simulink model "buildover_fullstatemachine"  (R2023a)
settings: Solver=FixedStepDiscrete  StartTime=0.0  StopTime=inf  FixedStep=0.001  RelTol=1e-3  EnableMultiTasking=on
undefined symbols (not defined in the file): dev, DiscIntNeverNeededParam, Main, output, pwm_output0, timestamp
libraries: simulink x15, px4uORBlib x7, robotcorelib x2, dspsigops x2, px4lib x1, px4Sensorslib x1, sharedtransform x1
settings Model: ExtModeTrigDuration=10  Creator=Kristan  LastModifiedBy=Kristan
settings SolverCC: PositivePriorityOrder=on  AutoInsertRateTranBlk=on
settings OptimizationCC: StrengthReduction=on  MemcpyThreshold=256  PassReuseOutputArgsAs=Individual arguments  ZeroExternalMemoryAtStartup=off  ZeroInternalMemoryAtStartup=off  MaxStackSize=128  OptimizeBlockOrder=speed  OptimizationPriority=Speed  OptimizationCustomize=off  MultiThreadedLoops=on  EfficientTunableParamExpr=on
settings DebuggingCC: ParameterTunabilityLossMsg=error  UnderSpecifiedDimensionMsg=warning
settings HardwareCC: ProdBitPerPointer=32  ProdBitPerSizeT=32  ProdBitPerPtrDiffT=32  ProdLargestAtomicInteger=Long  ProdLargestAtomicFloat=Double  ProdWordSize=32  ProdLongLongMode=on  ProdHWDeviceType=ARM Compatible->ARM Cortex
settings SFSimCC: MATLABDynamicMemAlloc=off  SimTargetLang=C++
settings RTWCC: Description=Embedded Coder  SystemTargetFile=ert.tlc  HardwareBoard=PX4 Pixhawk 6x  TLCOptions="-aInlineSetEventsForThisBaseRateFcn=TLC_FALSE -aSuppressMultiTaskScheduler=TLC_FALSE  -aRateBasedStepFcn=0"  TemplateMakefile=ert_default_tmf  GenerateReport=on  Toolchain=GNU Tools for PX4 Autopilots  LaunchReport=on  CodeProfilingSaveOptions=AllData  TargetLang=C++  GenerateCodeMetricsReport=on
settings CodeAppCC: GenerateComments=off  IgnoreCustomStorageClasses=off  OperatorAnnotations=on  SimulinkDataObjDesc=on  SFDataObjDesc=on  SimulinkBlockComments=off
settings ERTTargetCC: ExtModeTransport=3  ExtModeStaticAlloc=on  ExtModeStaticAllocSize=1024  ExtModeMexFile=ext_xcp  ExtModeIntrfLevel=Level2 - Open

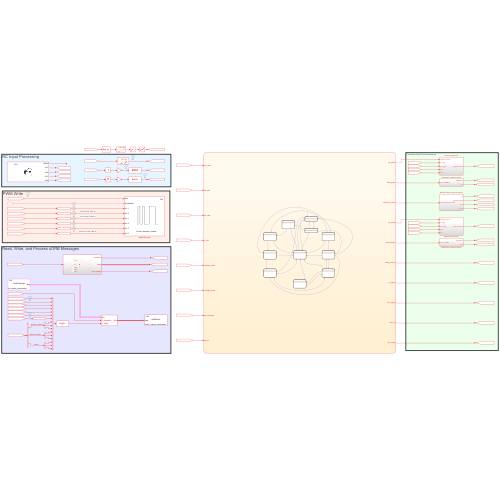
[thumbnail: Simulink's stored preview of the top-level diagram]
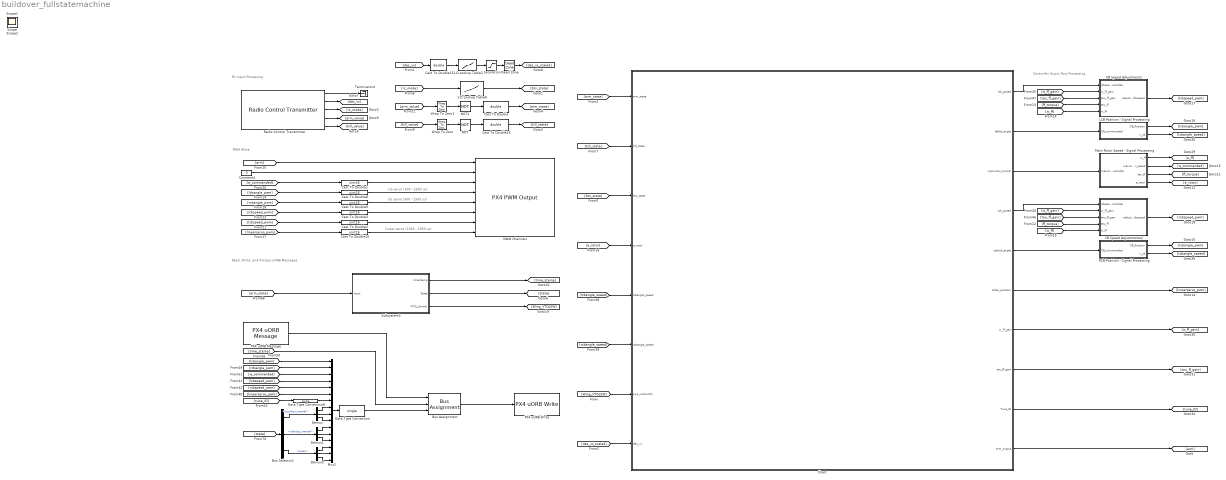
== system buildover_fullstatemachine ==
  note: Controller Ouput Post Processing
  note: PWM Write
  note: RC Input Processing
  note: Read, Write, and Process uORB Messages
  note: rcb servo (500 - 2500 us)
  note: lcb servo (500 - 2500 us)
  note: linear servo (1050 - 1950 us)
  1-D Lookup Table1 : Lookup_n-D  NumberOfTableDimensions=1  BreakpointsForDimension1=linspace(982,2006,2)  Table=linspace(-5,5,2)  InternalRulePriority=Speed  RndMeth=Simplest
  1-D Lookup Table6 : Lookup_n-D  NumberOfTableDimensions=1  BreakpointsForDimension1=[0, 1050, 1150, 1350, 1515, 1660, 1850]  Table=[1,2,3,4,5,6,7]  InterpMethod=Flat  InternalRulePriority=Speed  RndMeth=Simplest
  Bus Assignment : BusAssignment  AssignedSignals=timestamp,output
  Bus Selector1 : BusSelector  OutputSignals=position_inertial,velocity_inertial,euler
  CB Speed Adjustments : Subsystem
  CB Speed Adjustments2 : Subsystem
  Cast To Double : DataTypeConversion  OutDataTypeStr=double  SaturateOnIntegerOverflow=off  RndMeth=Floor
  Cast To Double{1..3,8..10} (6 alike) : DataTypeConversion  OutDataTypeStr=uint16  SaturateOnIntegerOverflow=off  RndMeth=Floor
  Cast To Double15 : DataTypeConversion  OutDataTypeStr=double  SaturateOnIntegerOverflow=off  RndMeth=Floor
  Cast To Double16 : DataTypeConversion  OutDataTypeStr=double  SaturateOnIntegerOverflow=off  RndMeth=Floor
  Chart : Stateflow chart  TreatAsAtomicUnit=on
  Constant4 : Constant  Value=0  OutDataTypeStr=boolean
  Data Type Conversion : DataTypeConversion  OutDataTypeStr=single  SaturateOnIntegerOverflow=off  RndMeth=Floor
  Data Type Conversion8 : DataTypeConversion  OutDataTypeStr=double  SaturateOnIntegerOverflow=off  RndMeth=Floor
  Dead Zone : DeadZone  LowerValue=-0.1  UpperValue=0.1
  Demux : Demux  Outputs=3
  Demux1 : Demux  Outputs=3
  Demux3 : Demux  Outputs=3
  LCB Position - Signal Processing : Subsystem
  MAIN Channels : px4lib/PX4 PWM Output  pwmDevice=Main (/dev/pwm_output0)  pwmChannel1_=on  pwmChannel2_=on  pwmChannel3_=on  pwmChannel4_=on  pwmChannel5_=on  pwmChannel6_=on  pwmChannel7_=off  pwmChannel8_=off  forceTerminateFailsafe=off  outputErrorStatus=off
  Main Rotor Speed - Signal Processing : Subsystem
  Mux2 : Mux  Inputs=16
  NOT : Logic  Operator=NOT  IconShape=distinctive  AllPortsSameDT=off  OutDataTypeStr=boolean
  NOT1 : Logic  Operator=NOT  IconShape=distinctive  AllPortsSameDT=off  OutDataTypeStr=boolean
  PX4 uORB Message : px4uORBlib/PX4 uORB Message  uORBTopic=actuator_outputs_commanded  SampleTime=inf  selectInstance=actuator_outputs_commanded
  PX4 uORB Write : px4uORBlib/PX4 uORB Write  uORBTopic=actuator_outputs_commanded  selectInstance=actuator_outputs_commanded  MessageQueueLen=1
  RCB Position - Signal Processing : Subsystem
  Radio Control Transmitter : px4Sensorslib/Radio Control Transmitter  channel1=off  channel2=off  channel3=on  channel4=off  channel5=off  channel6=on  channel7=on  channel8=on  channel_count=off  rssi=off  rc_input_source=off  timestamp_last_signal=off  time_stamp=off  sampleTime=-1  BlockingMode=off  BlockTimeout=5
  Saturation : Saturate  UpperLimit=5  LowerLimit=-5
  Subsystem3 : Subsystem
  Terminator4 : Terminator
  Wrap To Zero : simulink/Discontinuities/Wrap To Zero  Threshold=1500
  Wrap To Zero1 : simulink/Discontinuities/Wrap To Zero  Threshold=1500
  Scope : Scope
  Scope1 : Scope
  Scope2 : Scope
  wires:
  Radio Control Transmitter/5 -> [kill_value]
  Radio Control Transmitter/3 -> [rc_mode]
  Radio Control Transmitter/4 -> [arm_value]
  [btn_state] -> Chart/3(btn_state)
  [arm_state] -> Chart/1(arm_state)
  [kill_state] -> Chart/2(kill_state)
  [a_rotor] -> Chart/4(a_rotor)
  Chart/6(slider_position) -> [linearservo_pwm]
  Radio Control Transmitter/1 -> Terminator4/1
  1-D Lookup Table6/1 -> [btn_state]
  [arm_value] -> Wrap To Zero1/1
  Wrap To Zero1/1 -> NOT1/1
  [kill_value] -> Wrap To Zero/1
  [rc_mode] -> 1-D Lookup Table6/1
  Wrap To Zero/1 -> NOT/1
  Cast To Double16/1 -> [kill_state]
  NOT/1 -> Cast To Double16/1
  NOT1/1 -> Cast To Double/1
  Chart/7(w_ff_gain) -> [w_ff_gain]
  Chart/8(tau_ff_gain) -> [tau_ff_gain]
  Chart/3(mainrotor_control) -> Main Rotor Speed - Signal Processing/1(mainmotor_speed_controller)
  Main Rotor Speed - Signal Processing/1(w_ff) -> [w_ff]
  Main Rotor Speed - Signal Processing/2(mainmotor_speed) -> [w_commanded]
  Main Rotor Speed - Signal Processing/3(tau_ff) -> [ff_torque]
  Main Rotor Speed - Signal Processing/4(a_rotor) -> [a_rotor]
  Chart/1(lcb_speed) -> CB Speed Adjustments/1(lcbspeed_controller)
  [w_ff_gain] -> CB Speed Adjustments/2(w_ff_gain)
  [tau_ff_gain] -> CB Speed Adjustments/3(tau_ff_gain)
  [ff_torque] -> CB Speed Adjustments/4(tau_ff)
  [w_ff] -> CB Speed Adjustments/5(w_ff)
  Chart/4(rcb_speed) -> CB Speed Adjustments2/1(rcbspeed_controller)
  [w_ff_gain] -> CB Speed Adjustments2/2(w_ff_gain)
  [tau_ff_gain] -> CB Speed Adjustments2/3(tau_ff_gain)
  [ff_torque] -> CB Speed Adjustments2/4(tau_ff)
  [w_ff] -> CB Speed Adjustments2/5(w_ff)
  Chart/9(Tune_ID) -> [tune_ID]
  Chart/2(leftcb_angle) -> LCB Position - Signal Processing/1(CB_commanded)
  LCB Position - Signal Processing/1(CB_Position) -> [lcbangle_pwm]
  LCB Position - Signal Processing/2(v_cb) -> [lcbangle_speed]
  Chart/5(rightcb_angle) -> RCB Position - Signal Processing/1(CB_commanded)
  RCB Position - Signal Processing/1(CB_Position) -> [rcbangle_pwm]
  RCB Position - Signal Processing/2(v_cb) -> [rcbangle_speed]
  [lcbangle_speed] -> Chart/5(lcbangle_speed)
  [rcbangle_speed] -> Chart/6(rcbangle_speed)
  Cast To Double/1 -> [arm_state]
  PX4 uORB Message/1 -> Bus Assignment/1
  Bus Assignment/1 -> PX4 uORB Write/1
  [tune_ID] -> Data Type Conversion8/1
  Mux2/1 -> Data Type Conversion/1
  [rcbangle_pwm] -> Mux2/2
  [lcbangle_pwm] -> Mux2/1
  Chart/10(arm_output) -> [arm]
  [time_stamp] -> Bus Assignment/2
  CB Speed Adjustments/1(adjusted_lcbspeed) -> [lcbspeed_pwm]
  CB Speed Adjustments2/1(adjusted_rcbspeed) -> [rcbspeed_pwm]
  Subsystem3/2(State) -> [state]
  [arm_state] -> Subsystem3/1(Input)
  Subsystem3/1(timestamp) -> [time_stamp]
  [state] -> Bus Selector1/1
  Bus Selector1/2 -> Demux1/1  "<velocity_inertial>"
  Bus Selector1/3 -> Demux3/1  "<euler>"
  Bus Selector1/1 -> Demux/1  "<position_inertial>"
  Data Type Conversion/1 -> Bus Assignment/3
  Cast To Double8/1 -> MAIN Channels/4
  Cast To Double10/1 -> MAIN Channels/8
  Cast To Double2/1 -> MAIN Channels/7
  Cast To Double3/1 -> MAIN Channels/6
  Cast To Double1/1 -> MAIN Channels/3
  Cast To Double9/1 -> MAIN Channels/5
  [w_commanded] -> Cast To Double1/1
  Constant4/1 -> MAIN Channels/2
  [lcbspeed_pwm] -> Cast To Double2/1
  [rcbangle_pwm] -> Cast To Double9/1
  [rcbspeed_pwm] -> Cast To Double3/1
  [arm] -> MAIN Channels/1
  [linearservo_pwm] -> Cast To Double10/1
  [lcbangle_pwm] -> Cast To Double8/1
  [w_commanded] -> Mux2/3
  [lcbspeed_pwm] -> Mux2/4
  [rcbspeed_pwm] -> Mux2/5
  [linearservo_pwm] -> Mux2/6
  Data Type Conversion8/1 -> Mux2/7
  Demux3/3 -> Mux2/16
  Demux3/2 -> Mux2/15
  Demux3/1 -> Mux2/14
  Demux1/3 -> Mux2/13
  Demux1/2 -> Mux2/12
  Demux1/1 -> Mux2/11
  Demux/3 -> Mux2/10
  Demux/2 -> Mux2/9
  Demux/1 -> Mux2/8
  Subsystem3/3(VTOL_Switch) -> [Wing_VTOLSW]
  [Wing_VTOLSW] -> Chart/7(px4_vtolswitch)
  Radio Control Transmitter/2 -> [des_vx]
  Dead Zone/1 -> [des_vx_scaled]
  Saturation/1 -> Dead Zone/1
  1-D Lookup Table1/1 -> Saturation/1
  Cast To Double15/1 -> 1-D Lookup Table1/1
  [des_vx] -> Cast To Double15/1
  [des_vx_scaled] -> Chart/8(des_vx)

== system buildover_fullstatemachine/CB Speed Adjustments ==
  lcbspeed_controller : Inport
  w_ff_gain : Inport  Port=2
  tau_ff_gain : Inport  Port=3
  tau_ff : Inport  Port=4
  w_ff : Inport  Port=5
  1-D Lookup Table4 : Lookup_n-D  NumberOfTableDimensions=1  BreakpointsForDimension1=linspace(0,3300,2)  Table=linspace(1000,2000,2)  InternalRulePriority=Speed  RndMeth=Simplest
  Add1 : Sum
  Constant2 : Constant  Value=0  OutDataTypeStr=double
  Gain11 : Gain  Gain=0.018
  Gain7 : Gain  Gain=1600
  Product : Product
  Product2 : Product
  Saturation : Saturate  UpperLimit=2000  LowerLimit=1000
  Square1 : Math  Operator=square
  Sum4 : Sum  Inputs=|++
  Sum5 : Sum  Inputs=|++
  adjusted_lcbspeed : Outport
  wires:
  w_ff/1 -> Square1/1
  w_ff_gain/1 -> Product/1
  Product/1 -> Sum4/2
  tau_ff_gain/1 -> Product2/1
  Gain11/1 -> Product/2
  Square1/1 -> Gain11/1
  Product2/1 -> Sum5/2
  Sum4/1 -> 1-D Lookup Table4/1
  tau_ff/1 -> Product2/2
  Sum5/1 -> Sum4/1
  Saturation/1 -> adjusted_lcbspeed/1
  1-D Lookup Table4/1 -> Saturation/1
  Constant2/1 -> Add1/1
  Gain7/1 -> Add1/2
  lcbspeed_controller/1 -> Gain7/1
  Add1/1 -> Sum5/1

== system buildover_fullstatemachine/CB Speed Adjustments2 ==
  rcbspeed_controller : Inport
  w_ff_gain : Inport  Port=2
  tau_ff_gain : Inport  Port=3
  tau_ff : Inport  Port=4
  w_ff : Inport  Port=5
  1-D Lookup Table4 : Lookup_n-D  NumberOfTableDimensions=1  BreakpointsForDimension1=linspace(0,3300,2)  Table=linspace(1000,2000,2)  InternalRulePriority=Speed  RndMeth=Simplest
  Add1 : Sum
  Constant2 : Constant  Value=0  OutDataTypeStr=double
  Gain11 : Gain  Gain=0.018
  Gain6 : Gain  Gain=1600
  Product : Product
  Product2 : Product
  Saturation1 : Saturate  UpperLimit=2000  LowerLimit=1000
  Square1 : Math  Operator=square
  Sum4 : Sum  Inputs=|++
  Sum5 : Sum  Inputs=|++
  adjusted_rcbspeed : Outport
  wires:
  w_ff/1 -> Square1/1
  Sum5/1 -> Sum4/1
  w_ff_gain/1 -> Product/1
  Product/1 -> Sum4/2
  tau_ff_gain/1 -> Product2/1
  Gain11/1 -> Product/2
  Square1/1 -> Gain11/1
  Product2/1 -> Sum5/2
  tau_ff/1 -> Product2/2
  1-D Lookup Table4/1 -> Saturation1/1
  Sum4/1 -> 1-D Lookup Table4/1
  Saturation1/1 -> adjusted_rcbspeed/1
  Constant2/1 -> Add1/1
  Gain6/1 -> Add1/2
  Add1/1 -> Sum5/1
  rcbspeed_controller/1 -> Gain6/1

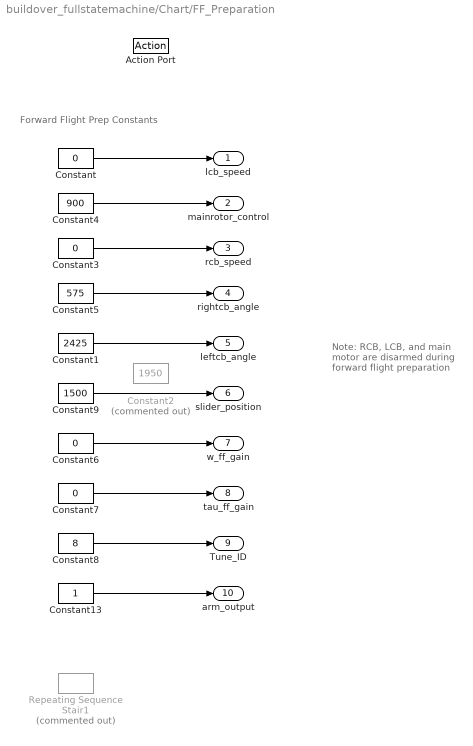
== system buildover_fullstatemachine/Chart/FF_Preparation ==
  note: Note: RCB, LCB, and main motor are disarmed during forward flight preparation
  note: Forward Flight Prep Constants
  Action Port : ActionPort
      settings: CopyFcn=Stateflow.SLINSF.SimulinkMan.removeBlockPreDeleteFcn  PreDeleteFcn=Stateflow.SLINSF.SimulinkMan.unsafePredeleteFcn
  Constant{,3,6..7} (4 alike) : Constant  Value=0  OutDataTypeStr=double
  Constant1 : Constant  Value=2425  OutDataTypeStr=double
  Constant13 : Constant  OutDataTypeStr=boolean
  Constant2 : Constant  Commented=on  Value=1950  OutDataTypeStr=double
  Constant4 : Constant  Value=900  OutDataTypeStr=double
  Constant5 : Constant  Value=575  OutDataTypeStr=double
  Constant8 : Constant  Value=8  OutDataTypeStr=double
  Constant9 : Constant  Value=1500  OutDataTypeStr=double
  Repeating Sequence Stair1 : simulink/Sources/Repeating Sequence Stair  Commented=on  OutValues=[1000 0 1000 0 1000 0 0 0 0 0 0 0 0 0 0 0 0 0 0].'  tsamp=-1  OutMin=[]  OutMax=[]  OutDataTypeStr=uint16  OutputDataTypeScalingMode=uint16  OutDataType=fixdt(0,8)  ConRadixGroup=Best Precision: Vector-wise  OutScaling=2^-12
  lcb_speed : Outport
  mainrotor_control : Outport  Port=2
  rcb_speed : Outport  Port=3
  rightcb_angle : Outport  Port=4
  leftcb_angle : Outport  Port=5
  slider_position : Outport  Port=6
  w_ff_gain : Outport  Port=7
  tau_ff_gain : Outport  Port=8
  Tune_ID : Outport  Port=9
  arm_output : Outport  Port=10
  wires:
  Constant3/1 -> rcb_speed/1
  Constant4/1 -> mainrotor_control/1
  Constant/1 -> lcb_speed/1
  Constant6/1 -> w_ff_gain/1
  Constant7/1 -> tau_ff_gain/1
  Constant13/1 -> arm_output/1
  Constant8/1 -> Tune_ID/1
  Constant1/1 -> leftcb_angle/1
  Constant5/1 -> rightcb_angle/1
  Constant9/1 -> slider_position/1

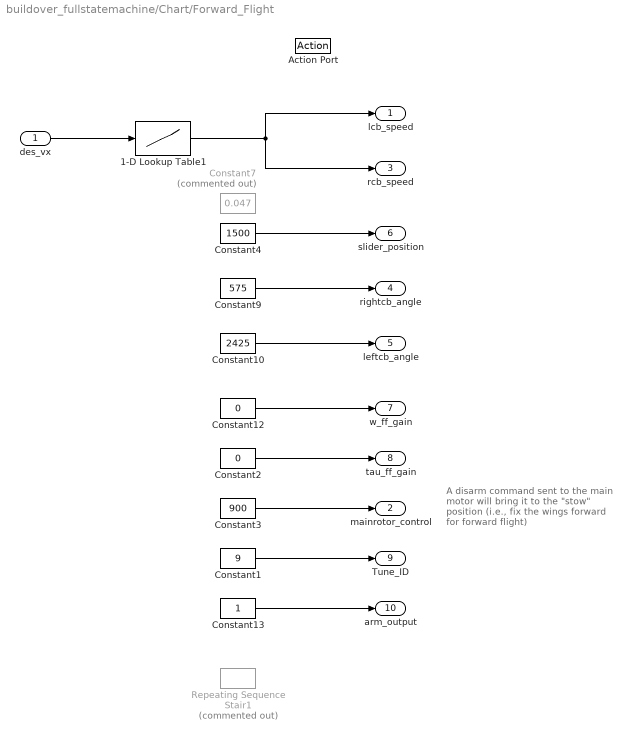
== system buildover_fullstatemachine/Chart/Forward_Flight ==
  note: A disarm command sent to the main motor will bring it to the "stow" position (i.e., fix the wings forward for forward flight)
  des_vx : Inport
  Action Port : ActionPort
      settings: CopyFcn=Stateflow.SLINSF.SimulinkMan.removeBlockPreDeleteFcn  PreDeleteFcn=Stateflow.SLINSF.SimulinkMan.unsafePredeleteFcn
  1-D Lookup Table1 : Lookup_n-D  NumberOfTableDimensions=1  BreakpointsForDimension1=linspace(-5,5,2)  Table=linspace(-0.5,0.5,2)  InternalRulePriority=Speed  RndMeth=Simplest
  Constant1 : Constant  Value=9  OutDataTypeStr=double
  Constant10 : Constant  Value=2425  OutDataTypeStr=double
  Constant12 : Constant  Value=0  OutDataTypeStr=double
  Constant13 : Constant  OutDataTypeStr=boolean
  Constant2 : Constant  Value=0  OutDataTypeStr=double
  Constant3 : Constant  Value=900  OutDataTypeStr=double
  Constant4 : Constant  Value=1500  OutDataTypeStr=double
  Constant7 : Constant  Commented=on  Value=0.047  OutDataTypeStr=double
  Constant9 : Constant  Value=575  OutDataTypeStr=double
  Repeating Sequence Stair1 : simulink/Sources/Repeating Sequence Stair  Commented=on  OutValues=[1000 0 1000 0 1000 0 1000 0 1000 0 1000 0 0 0 0 0 0 0 0].'  tsamp=-1  OutMin=[]  OutMax=[]  OutDataTypeStr=uint16  OutputDataTypeScalingMode=uint16  OutDataType=fixdt(0,8)  ConRadixGroup=Best Precision: Vector-wise  OutScaling=2^-12
  lcb_speed : Outport
  mainrotor_control : Outport  Port=2
  rcb_speed : Outport  Port=3
  rightcb_angle : Outport  Port=4
  leftcb_angle : Outport  Port=5
  slider_position : Outport  Port=6
  w_ff_gain : Outport  Port=7
  tau_ff_gain : Outport  Port=8
  Tune_ID : Outport  Port=9
  arm_output : Outport  Port=10
  wires:
  Constant12/1 -> w_ff_gain/1
  Constant2/1 -> tau_ff_gain/1
  Constant3/1 -> mainrotor_control/1
  Constant13/1 -> arm_output/1
  Constant9/1 -> rightcb_angle/1
  Constant10/1 -> leftcb_angle/1
  1-D Lookup Table1/1 -> rcb_speed/1, lcb_speed/1
  des_vx/1 -> 1-D Lookup Table1/1
  Constant1/1 -> Tune_ID/1
  Constant4/1 -> slider_position/1

== system buildover_fullstatemachine/Chart/Kill ==
  Action Port : ActionPort
      settings: CopyFcn=Stateflow.SLINSF.SimulinkMan.removeBlockPreDeleteFcn  PreDeleteFcn=Stateflow.SLINSF.SimulinkMan.unsafePredeleteFcn
  Constant : Constant  Value=0  OutDataTypeStr=double
  Constant1 : Constant  Value=0  OutDataTypeStr=boolean
  Constant13 : Constant  Value=10  OutDataTypeStr=double
  Repeating Sequence Stair1 : simulink/Sources/Repeating Sequence Stair  Commented=on  OutValues=[1000 0 1000 0 1000 0 1000 0 1000 0 1000 0 1000 0 1000 0 1000 0].'  tsamp=-1  OutMin=[]  OutMax=[]  OutDataTypeStr=uint16  OutputDataTypeScalingMode=uint16  OutDataType=fixdt(0,8)  ConRadixGroup=Best Precision: Vector-wise  OutScaling=2^-12
  lcb_speed : Outport
  mainrotor_control : Outport  Port=2
  rcb_speed : Outport  Port=3
  rightcb_angle : Outport  Port=4
  leftcb_angle : Outport  Port=5
  slider_position : Outport  Port=6
  w_ff_gain : Outport  Port=7
  tau_ff_gain : Outport  Port=8
  Tune_ID : Outport  Port=9
  arm_output : Outport  Port=10
  wires:
  Constant/1 -> lcb_speed/1, mainrotor_control/1, rcb_speed/1, rightcb_angle/1, leftcb_angle/1, slider_position/1, w_ff_gain/1, tau_ff_gain/1
  Constant1/1 -> arm_output/1
  Constant13/1 -> Tune_ID/1

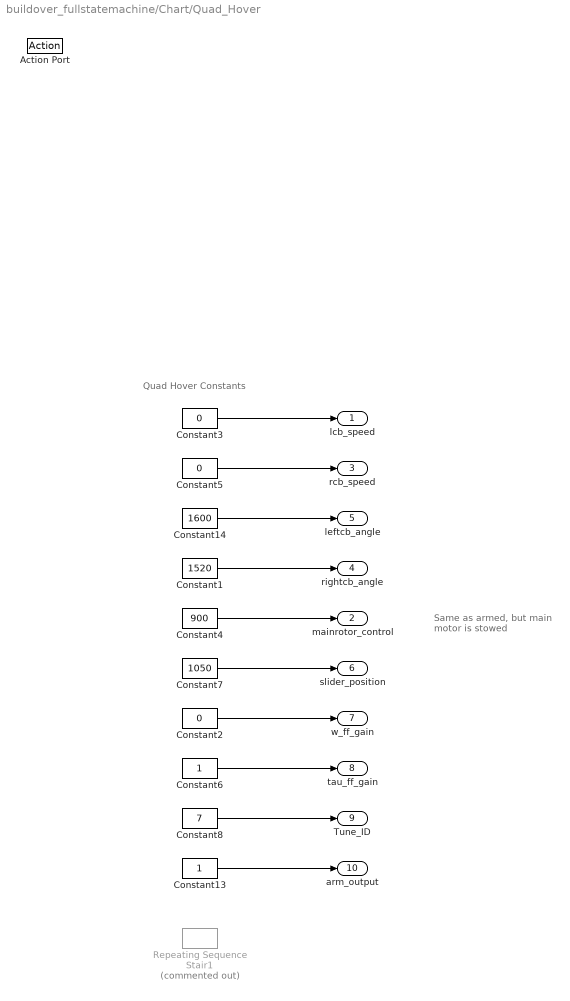
== system buildover_fullstatemachine/Chart/Quad_Hover ==
  note: Same as armed, but main motor is stowed
  note: Quad Hover Constants
  Action Port : ActionPort
      settings: CopyFcn=Stateflow.SLINSF.SimulinkMan.removeBlockPreDeleteFcn  PreDeleteFcn=Stateflow.SLINSF.SimulinkMan.unsafePredeleteFcn
  Constant1 : Constant  Value=1520  OutDataTypeStr=double
  Constant13 : Constant  OutDataTypeStr=boolean
  Constant14 : Constant  Value=1600  OutDataTypeStr=double
  Constant2 : Constant  Value=0  OutDataTypeStr=double
  Constant3 : Constant  Value=0  OutDataTypeStr=double
  Constant4 : Constant  Value=900  OutDataTypeStr=double
  Constant5 : Constant  Value=0  OutDataTypeStr=double
  Constant6 : Constant  OutDataTypeStr=double
  Constant7 : Constant  Value=1050  OutDataTypeStr=double
  Constant8 : Constant  Value=7  OutDataTypeStr=double
  Repeating Sequence Stair1 : simulink/Sources/Repeating Sequence Stair  Commented=on  OutValues=[1000 0 1000 0 0 0 0 0 0 0 0 0 0 0 0 0 0 0 0].'  tsamp=-1  OutMin=[]  OutMax=[]  OutDataTypeStr=uint16  OutputDataTypeScalingMode=uint16  OutDataType=fixdt(0,8)  ConRadixGroup=Best Precision: Vector-wise  OutScaling=2^-12
  lcb_speed : Outport
  mainrotor_control : Outport  Port=2
  rcb_speed : Outport  Port=3
  rightcb_angle : Outport  Port=4
  leftcb_angle : Outport  Port=5
  slider_position : Outport  Port=6
  w_ff_gain : Outport  Port=7
  tau_ff_gain : Outport  Port=8
  Tune_ID : Outport  Port=9
  arm_output : Outport  Port=10
  wires:
  Constant7/1 -> slider_position/1
  Constant4/1 -> mainrotor_control/1
  Constant2/1 -> w_ff_gain/1
  Constant6/1 -> tau_ff_gain/1
  Constant13/1 -> arm_output/1
  Constant1/1 -> rightcb_angle/1
  Constant14/1 -> leftcb_angle/1
  Constant3/1 -> lcb_speed/1
  Constant5/1 -> rcb_speed/1
  Constant8/1 -> Tune_ID/1

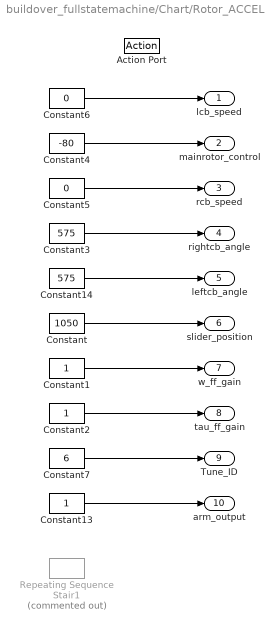
== system buildover_fullstatemachine/Chart/Rotor_ACCEL ==
  Action Port : ActionPort
      settings: CopyFcn=Stateflow.SLINSF.SimulinkMan.removeBlockPreDeleteFcn  PreDeleteFcn=Stateflow.SLINSF.SimulinkMan.unsafePredeleteFcn
  Constant : Constant  Value=1050  OutDataTypeStr=double
  Constant1 : Constant  OutDataTypeStr=double
  Constant13 : Constant  OutDataTypeStr=boolean
  Constant14 : Constant  Value=575  OutDataTypeStr=double
  Constant2 : Constant  OutDataTypeStr=double
  Constant3 : Constant  Value=575  OutDataTypeStr=double
  Constant4 : Constant  Value=-80  OutDataTypeStr=double
  Constant5 : Constant  Value=0  OutDataTypeStr=double
  Constant6 : Constant  Value=0  OutDataTypeStr=double
  Constant7 : Constant  Value=6  OutDataTypeStr=double
  Repeating Sequence Stair1 : simulink/Sources/Repeating Sequence Stair  Commented=on  OutValues=[1000 0 1000 0 1000 0 0 0 0 0 0 0 0 0 0 0 0 0 0].'  tsamp=-1  OutMin=[]  OutMax=[]  OutDataTypeStr=uint16  OutputDataTypeScalingMode=uint16  OutDataType=fixdt(0,8)  ConRadixGroup=Best Precision: Vector-wise  OutScaling=2^-12
  lcb_speed : Outport
  mainrotor_control : Outport  Port=2
  rcb_speed : Outport  Port=3
  rightcb_angle : Outport  Port=4
  leftcb_angle : Outport  Port=5
  slider_position : Outport  Port=6
  w_ff_gain : Outport  Port=7
  tau_ff_gain : Outport  Port=8
  Tune_ID : Outport  Port=9
  arm_output : Outport  Port=10
  wires:
  Constant6/1 -> lcb_speed/1
  Constant4/1 -> mainrotor_control/1
  Constant5/1 -> rcb_speed/1
  Constant14/1 -> leftcb_angle/1
  Constant3/1 -> rightcb_angle/1
  Constant/1 -> slider_position/1
  Constant1/1 -> w_ff_gain/1
  Constant2/1 -> tau_ff_gain/1
  Constant13/1 -> arm_output/1
  Constant7/1 -> Tune_ID/1

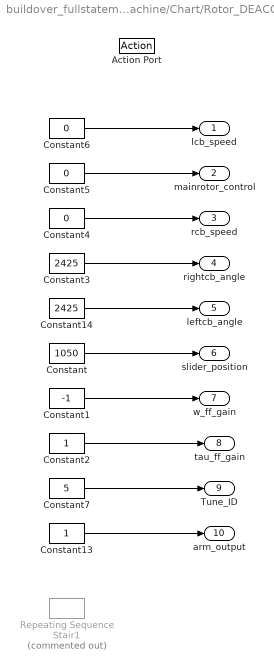
== system buildover_fullstatemachine/Chart/Rotor_DEACCEL ==
  Action Port : ActionPort
      settings: CopyFcn=Stateflow.SLINSF.SimulinkMan.removeBlockPreDeleteFcn  PreDeleteFcn=Stateflow.SLINSF.SimulinkMan.unsafePredeleteFcn
  Constant : Constant  Value=1050  OutDataTypeStr=double
  Constant1 : Constant  Value=-1  OutDataTypeStr=double
  Constant13 : Constant  OutDataTypeStr=boolean
  Constant14 : Constant  Value=2425  OutDataTypeStr=double
  Constant2 : Constant  OutDataTypeStr=double
  Constant3 : Constant  Value=2425  OutDataTypeStr=double
  Constant4 : Constant  Value=0  OutDataTypeStr=double
  Constant5 : Constant  Value=0  OutDataTypeStr=double
  Constant6 : Constant  Value=0  OutDataTypeStr=double
  Constant7 : Constant  Value=5  OutDataTypeStr=double
  Repeating Sequence Stair1 : simulink/Sources/Repeating Sequence Stair  Commented=on  OutValues=[1000 0 1000 0 1000 0 0 0 0 0 0 0 0 0 0 0 0 0 0].'  tsamp=-1  OutMin=[]  OutMax=[]  OutDataTypeStr=uint16  OutputDataTypeScalingMode=uint16  OutDataType=fixdt(0,8)  ConRadixGroup=Best Precision: Vector-wise  OutScaling=2^-12
  lcb_speed : Outport
  mainrotor_control : Outport  Port=2
  rcb_speed : Outport  Port=3
  rightcb_angle : Outport  Port=4
  leftcb_angle : Outport  Port=5
  slider_position : Outport  Port=6
  w_ff_gain : Outport  Port=7
  tau_ff_gain : Outport  Port=8
  Tune_ID : Outport  Port=9
  arm_output : Outport  Port=10
  wires:
  Constant6/1 -> lcb_speed/1
  Constant5/1 -> mainrotor_control/1
  Constant4/1 -> rcb_speed/1
  Constant14/1 -> leftcb_angle/1
  Constant3/1 -> rightcb_angle/1
  Constant/1 -> slider_position/1
  Constant1/1 -> w_ff_gain/1
  Constant2/1 -> tau_ff_gain/1
  Constant13/1 -> arm_output/1
  Constant7/1 -> Tune_ID/1

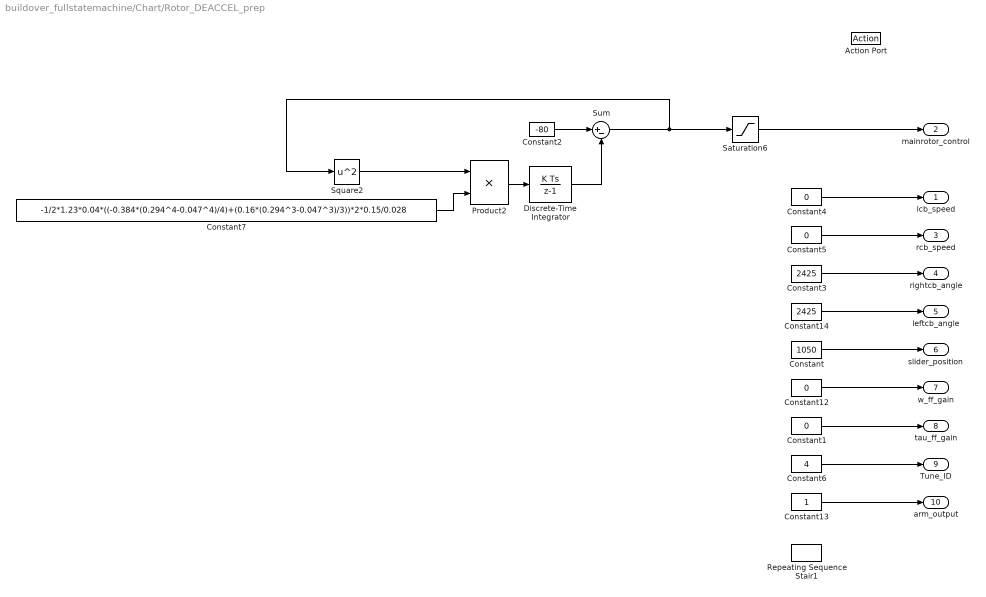
== system buildover_fullstatemachine/Chart/Rotor_DEACCEL_prep ==
  Action Port : ActionPort
      settings: CopyFcn=Stateflow.SLINSF.SimulinkMan.removeBlockPreDeleteFcn  PreDeleteFcn=Stateflow.SLINSF.SimulinkMan.unsafePredeleteFcn
  Constant : Constant  Value=1050  OutDataTypeStr=double
  Constant{1,4..5,12} (4 alike) : Constant  Value=0  OutDataTypeStr=double
  Constant13 : Constant  OutDataTypeStr=boolean
  Constant14 : Constant  Value=2425  OutDataTypeStr=double
  Constant2 : Constant  Value=-80  OutDataTypeStr=double
  Constant3 : Constant  Value=2425  OutDataTypeStr=double
  Constant6 : Constant  Value=4  OutDataTypeStr=double
  Constant7 : Constant  Value=-1/2*1.23*0.04*((-0.384*(0.294^4-0.047^4)/4)+(0.16*(0.294^3-0.047^3)/3))*2*0.15/0.028  OutDataTypeStr=double
  Discrete-Time Integrator : DiscreteIntegrator  SampleTime=-1  LimitOutput=on  UpperSaturationLimit=0  LowerSaturationLimit=-12  ICPrevOutput=DiscIntNeverNeededParam  ICPrevScaledInput=DiscIntNeverNeededParam
  Product2 : Product
  Repeating Sequence Stair1 : simulink/Sources/Repeating Sequence Stair  OutValues=[1000 0 1000 0 1000 0 0 0 0 0 0 0 0 0 0 0 0 0 0].'  tsamp=-1  OutMin=[]  OutMax=[]  OutDataTypeStr=uint16  OutputDataTypeScalingMode=uint16  OutDataType=fixdt(0,8)  ConRadixGroup=Best Precision: Vector-wise  OutScaling=2^-12
  Saturation6 : Saturate  UpperLimit=0  LowerLimit=-125
  Square2 : Math  Operator=square
  Sum : Sum  Inputs=|+-
  lcb_speed : Outport
  mainrotor_control : Outport  Port=2
  rcb_speed : Outport  Port=3
  rightcb_angle : Outport  Port=4
  leftcb_angle : Outport  Port=5
  slider_position : Outport  Port=6
  w_ff_gain : Outport  Port=7
  tau_ff_gain : Outport  Port=8
  Tune_ID : Outport  Port=9
  arm_output : Outport  Port=10
  wires:
  Constant4/1 -> lcb_speed/1
  Saturation6/1 -> mainrotor_control/1
  Constant5/1 -> rcb_speed/1
  Constant14/1 -> leftcb_angle/1
  Constant3/1 -> rightcb_angle/1
  Constant/1 -> slider_position/1
  Constant12/1 -> w_ff_gain/1
  Constant1/1 -> tau_ff_gain/1
  Constant13/1 -> arm_output/1
  Product2/1 -> Discrete-Time Integrator/1
  Discrete-Time Integrator/1 -> Sum/2
  Constant7/1 -> Product2/2
  Square2/1 -> Product2/1
  Sum/1 -> Saturation6/1, Square2/1
  Constant2/1 -> Sum/1
  Constant6/1 -> Tune_ID/1

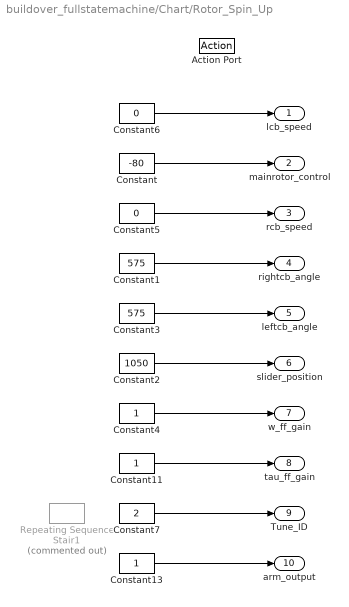
== system buildover_fullstatemachine/Chart/Rotor_Spin_Up ==
  Action Port : ActionPort
      settings: CopyFcn=Stateflow.SLINSF.SimulinkMan.removeBlockPreDeleteFcn  PreDeleteFcn=Stateflow.SLINSF.SimulinkMan.unsafePredeleteFcn
  Constant : Constant  Value=-80  OutDataTypeStr=double
  Constant1 : Constant  Value=575  OutDataTypeStr=double
  Constant11 : Constant  OutDataTypeStr=double
  Constant13 : Constant  OutDataTypeStr=boolean
  Constant2 : Constant  Value=1050  OutDataTypeStr=double
  Constant3 : Constant  Value=575  OutDataTypeStr=double
  Constant4 : Constant  OutDataTypeStr=double
  Constant5 : Constant  Value=0  OutDataTypeStr=double
  Constant6 : Constant  Value=0  OutDataTypeStr=double
  Constant7 : Constant  Value=2  OutDataTypeStr=double
  Repeating Sequence Stair1 : simulink/Sources/Repeating Sequence Stair  Commented=on  OutValues=[1000 0 1000 0 1000 0 1000 0 0 0 0 0 0 0 0 0 0 0 0].'  tsamp=-1  OutMin=[]  OutMax=[]  OutDataTypeStr=uint16  OutputDataTypeScalingMode=uint16  OutDataType=fixdt(0,8)  ConRadixGroup=Best Precision: Vector-wise  OutScaling=2^-12
  lcb_speed : Outport
  mainrotor_control : Outport  Port=2
  rcb_speed : Outport  Port=3
  rightcb_angle : Outport  Port=4
  leftcb_angle : Outport  Port=5
  slider_position : Outport  Port=6
  w_ff_gain : Outport  Port=7
  tau_ff_gain : Outport  Port=8
  Tune_ID : Outport  Port=9
  arm_output : Outport  Port=10
  wires:
  Constant6/1 -> lcb_speed/1
  Constant/1 -> mainrotor_control/1
  Constant5/1 -> rcb_speed/1
  Constant1/1 -> rightcb_angle/1
  Constant3/1 -> leftcb_angle/1
  Constant2/1 -> slider_position/1
  Constant4/1 -> w_ff_gain/1
  Constant11/1 -> tau_ff_gain/1
  Constant13/1 -> arm_output/1
  Constant7/1 -> Tune_ID/1

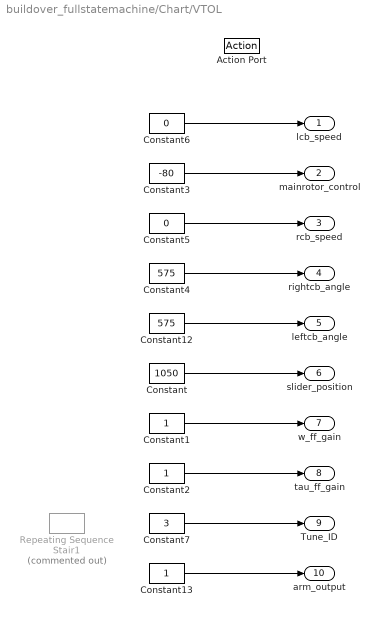
== system buildover_fullstatemachine/Chart/VTOL ==
  Action Port : ActionPort
      settings: CopyFcn=Stateflow.SLINSF.SimulinkMan.removeBlockPreDeleteFcn  PreDeleteFcn=Stateflow.SLINSF.SimulinkMan.unsafePredeleteFcn
  Constant : Constant  Value=1050  OutDataTypeStr=double
  Constant1 : Constant  OutDataTypeStr=double
  Constant12 : Constant  Value=575  OutDataTypeStr=double
  Constant13 : Constant  OutDataTypeStr=boolean
  Constant2 : Constant  OutDataTypeStr=double
  Constant3 : Constant  Value=-80  OutDataTypeStr=double
  Constant4 : Constant  Value=575  OutDataTypeStr=double
  Constant5 : Constant  Value=0  OutDataTypeStr=double
  Constant6 : Constant  Value=0  OutDataTypeStr=double
  Constant7 : Constant  Value=3  OutDataTypeStr=double
  Repeating Sequence Stair1 : simulink/Sources/Repeating Sequence Stair  Commented=on  OutValues=[1000 0 1000 0 1000 0 1000 0 0 0 0 0 0 0 0 0 0 0 0].'  tsamp=-1  OutMin=[]  OutMax=[]  OutDataTypeStr=uint16  OutputDataTypeScalingMode=uint16  OutDataType=fixdt(0,8)  ConRadixGroup=Best Precision: Vector-wise  OutScaling=2^-12
  lcb_speed : Outport
  mainrotor_control : Outport  Port=2
  rcb_speed : Outport  Port=3
  rightcb_angle : Outport  Port=4
  leftcb_angle : Outport  Port=5
  slider_position : Outport  Port=6
  w_ff_gain : Outport  Port=7
  tau_ff_gain : Outport  Port=8
  Tune_ID : Outport  Port=9
  arm_output : Outport  Port=10
  wires:
  Constant12/1 -> leftcb_angle/1
  Constant4/1 -> rightcb_angle/1
  Constant6/1 -> lcb_speed/1
  Constant3/1 -> mainrotor_control/1
  Constant5/1 -> rcb_speed/1
  Constant/1 -> slider_position/1
  Constant1/1 -> w_ff_gain/1
  Constant2/1 -> tau_ff_gain/1
  Constant13/1 -> arm_output/1
  Constant7/1 -> Tune_ID/1

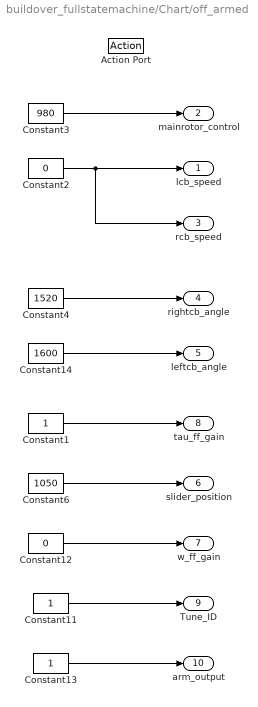
== system buildover_fullstatemachine/Chart/off_armed ==
  Action Port : ActionPort
      settings: CopyFcn=Stateflow.SLINSF.SimulinkMan.removeBlockPreDeleteFcn  PreDeleteFcn=Stateflow.SLINSF.SimulinkMan.unsafePredeleteFcn
  Constant1 : Constant  OutDataTypeStr=double
  Constant11 : Constant  OutDataTypeStr=double
  Constant12 : Constant  Value=0  OutDataTypeStr=double
  Constant13 : Constant  OutDataTypeStr=boolean
  Constant14 : Constant  Value=1600  OutDataTypeStr=double
  Constant2 : Constant  Value=0  OutDataTypeStr=double
  Constant3 : Constant  Value=980  OutDataTypeStr=double
  Constant4 : Constant  Value=1520  OutDataTypeStr=double
  Constant6 : Constant  Value=1050  OutDataTypeStr=double
  lcb_speed : Outport
  mainrotor_control : Outport  Port=2
  rcb_speed : Outport  Port=3
  rightcb_angle : Outport  Port=4
  leftcb_angle : Outport  Port=5
  slider_position : Outport  Port=6
  w_ff_gain : Outport  Port=7
  tau_ff_gain : Outport  Port=8
  Tune_ID : Outport  Port=9
  arm_output : Outport  Port=10
  wires:
  Constant6/1 -> slider_position/1
  Constant4/1 -> rightcb_angle/1
  Constant12/1 -> w_ff_gain/1
  Constant1/1 -> tau_ff_gain/1
  Constant2/1 -> rcb_speed/1, lcb_speed/1
  Constant3/1 -> mainrotor_control/1
  Constant11/1 -> Tune_ID/1
  Constant13/1 -> arm_output/1
  Constant14/1 -> leftcb_angle/1

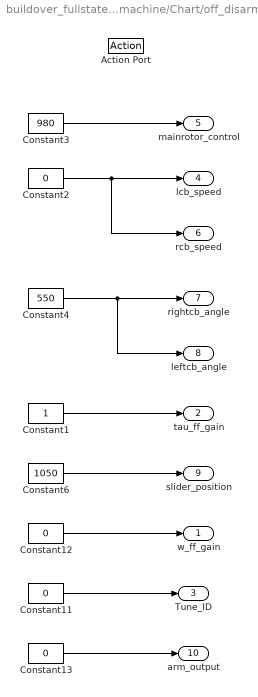
== system buildover_fullstatemachine/Chart/off_disarmed ==
  Action Port : ActionPort
      settings: CopyFcn=Stateflow.SLINSF.SimulinkMan.removeBlockPreDeleteFcn  PreDeleteFcn=Stateflow.SLINSF.SimulinkMan.unsafePredeleteFcn
  Constant1 : Constant  OutDataTypeStr=double
  Constant11 : Constant  Value=0  OutDataTypeStr=double
  Constant12 : Constant  Value=0  OutDataTypeStr=double
  Constant13 : Constant  Value=0  OutDataTypeStr=boolean
  Constant2 : Constant  Value=0  OutDataTypeStr=double
  Constant3 : Constant  Value=980  OutDataTypeStr=double
  Constant4 : Constant  Value=550  OutDataTypeStr=double
  Constant6 : Constant  Value=1050  OutDataTypeStr=double
  w_ff_gain : Outport
  tau_ff_gain : Outport  Port=2
  Tune_ID : Outport  Port=3
  lcb_speed : Outport  Port=4
  mainrotor_control : Outport  Port=5
  rcb_speed : Outport  Port=6
  rightcb_angle : Outport  Port=7
  leftcb_angle : Outport  Port=8
  slider_position : Outport  Port=9
  arm_output : Outport  Port=10
  wires:
  Constant12/1 -> w_ff_gain/1
  Constant1/1 -> tau_ff_gain/1
  Constant11/1 -> Tune_ID/1
  Constant3/1 -> mainrotor_control/1
  Constant4/1 -> leftcb_angle/1, rightcb_angle/1
  Constant6/1 -> slider_position/1
  Constant13/1 -> arm_output/1
  Constant2/1 -> rcb_speed/1, lcb_speed/1

== system buildover_fullstatemachine/LCB Position - Signal Processing ==
  CB_commanded : Inport
  Discrete Derivative : simulink/Discrete/Discrete Derivative  gainval=1.0  ICPrevScaledInput=0.0  OutMin=[]  OutMax=[]  OutDataType=fixdt(1, 16)  OutScaling=2^-10  DoSatur=off
  Memory : Memory
  Rate Limiter1 : RateLimiter  RisingSlewLimit=750  FallingSlewLimit=-750  SampleTimeMode=inherited
  CB_Position : Outport
  v_cb : Outport  Port=2
  wires:
  CB_commanded/1 -> Rate Limiter1/1
  Discrete Derivative/1 -> v_cb/1
  Memory/1 -> Discrete Derivative/1
  Rate Limiter1/1 -> Memory/1, CB_Position/1

== system buildover_fullstatemachine/Main Rotor Speed - Signal Processing ==
  mainmotor_speed_controller : Inport
  1-D Lookup Table5 : Lookup_n-D  NumberOfTableDimensions=1  BreakpointsForDimension1=linspace(0,638,2)  Table=linspace(1000,2000,2)  InternalRulePriority=Speed  RndMeth=Simplest
  Abs : Abs  SaturateOnIntegerOverflow=off
  Constant : Constant  Value=0  OutDataTypeStr=double
  Discrete Derivative : simulink/Discrete/Discrete Derivative  gainval=1.0  ICPrevScaledInput=0.0  OutMin=[]  OutMax=[]  OutDataType=fixdt(1, 16)  OutScaling=2^-10  DoSatur=off
  Gain : Gain  Gain=18.4  OutDataTypeStr=double  LockScale=on
  Memory : Memory
  Rate Limiter : RateLimiter  RisingSlewLimit=20  FallingSlewLimit=-20  SampleTimeMode=inherited
  Saturation5 : Saturate  UpperLimit=2000  LowerLimit=1000
  Saturation7 : Saturate  UpperLimit=0  LowerLimit=-60  OutDataTypeStr=double
  Switch : Switch  Criteria=u2 > Threshold  Threshold=250  SaturateOnIntegerOverflow=off  InputSameDT=off
  Switch1 : Switch  Criteria=u2 > Threshold  Threshold=250  SaturateOnIntegerOverflow=off  InputSameDT=off
  Unary Minus : UnaryMinus
  w_ff : Outport
  mainmotor_speed : Outport  Port=2
  tau_ff : Outport  Port=3
  a_rotor : Outport  Port=4
  wires:
  Memory/1 -> Saturation7/1
  Abs/1 -> Gain/1
  1-D Lookup Table5/1 -> Saturation5/1
  Gain/1 -> tau_ff/1
  [w_commanded] -> Switch/2, Switch/1
  Switch/1 -> mainmotor_speed/1
  Switch1/1 -> Memory/1
  mainmotor_speed_controller/1 -> [w_commanded], Switch1/2, Switch1/3
  Constant/1 -> Switch1/1
  Unary Minus/1 -> w_ff/1, 1-D Lookup Table5/1
  Saturation5/1 -> Switch/3
  Rate Limiter/1 -> Discrete Derivative/1, Unary Minus/1
  Saturation7/1 -> Rate Limiter/1
  Discrete Derivative/1 -> a_rotor/1, Abs/1

== system buildover_fullstatemachine/RCB Position - Signal Processing ==
  CB_commanded : Inport
  Discrete Derivative : simulink/Discrete/Discrete Derivative  gainval=1.0  ICPrevScaledInput=0.0  OutMin=[]  OutMax=[]  OutDataType=fixdt(1, 16)  OutScaling=2^-10  DoSatur=off
  Memory1 : Memory
  Rate Limiter1 : RateLimiter  RisingSlewLimit=750  FallingSlewLimit=-750  SampleTimeMode=inherited
  CB_Position : Outport
  v_cb : Outport  Port=2
  wires:
  CB_commanded/1 -> Rate Limiter1/1
  Discrete Derivative/1 -> v_cb/1
  Memory1/1 -> Discrete Derivative/1
  Rate Limiter1/1 -> CB_Position/1, Memory1/1

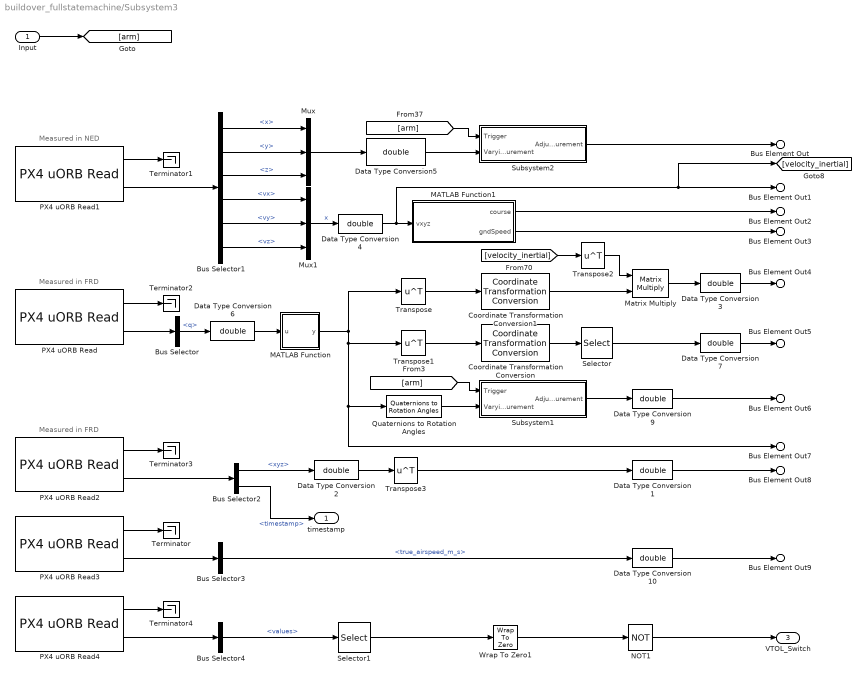
== system buildover_fullstatemachine/Subsystem3 ==
  note: Measured in FRD
  note: Measured in FRD
  note: Measured in NED
  Input : Inport
  Bus Selector : BusSelector  OutputSignals=q
  Bus Selector1 : BusSelector  OutputSignals=x,y,z,vx,vy,vz
  Bus Selector2 : BusSelector  OutputSignals=xyz,timestamp
  Bus Selector3 : BusSelector  OutputSignals=true_airspeed_m_s
  Bus Selector4 : BusSelector  OutputSignals=values
  Coordinate Transformation Conversion : robotcorelib/Coordinate Transformation Conversion  InputRepresentation=Quaternion  InputEulerSequence=ZYX  ShowTrVecInputPort=on  OutputRepresentation=Euler Angles  OutputEulerSequence=ZYX  ShowTrVecOutputPort=on  SimulateUsing=Interpreted execution
  Coordinate Transformation Conversion1 : robotcorelib/Coordinate Transformation Conversion  InputRepresentation=Quaternion  InputEulerSequence=ZYX  ShowTrVecInputPort=on  OutputRepresentation=Rotation Matrix  OutputEulerSequence=ZYX  ShowTrVecOutputPort=on  SimulateUsing=Interpreted execution
  Data Type Conversion{1..7,9..10} (9 alike) : DataTypeConversion  OutDataTypeStr=double  SaturateOnIntegerOverflow=off  RndMeth=Floor
  MATLAB Function : MATLAB Function  TreatAsAtomicUnit=on
  MATLAB Function1 : MATLAB Function  TreatAsAtomicUnit=on
  Matrix Multiply : Product  Multiplication=Matrix(*)
  Mux : Mux  Inputs=3
  Mux1 : Mux  Inputs=3
  NOT1 : Logic  Operator=NOT  IconShape=distinctive  AllPortsSameDT=off  OutDataTypeStr=boolean
  PX4 uORB Read : px4uORBlib/PX4 uORB Read  uORBTopic=vehicle_attitude  selectInstance=vehicle_attitude  SampleTime=-1  BlockingMode=off  BlockTimeout=1e-3
  PX4 uORB Read1 : px4uORBlib/PX4 uORB Read  uORBTopic=vehicle_local_position  selectInstance=vehicle_local_position  SampleTime=-1  BlockingMode=off  BlockTimeout=1e-3
  PX4 uORB Read2 : px4uORBlib/PX4 uORB Read  uORBTopic=vehicle_angular_velocity  selectInstance=vehicle_angular_velocity  SampleTime=-1  BlockingMode=off  BlockTimeout=1e-3
  PX4 uORB Read3 : px4uORBlib/PX4 uORB Read  uORBTopic=airspeed  selectInstance=airspeed  SampleTime=-1  BlockingMode=off  BlockTimeout=1e-3
  PX4 uORB Read4 : px4uORBlib/PX4 uORB Read  uORBTopic=input_rc  selectInstance=input_rc  SampleTime=-1  BlockingMode=off  BlockTimeout=1e-3
  Quaternions to Rotation Angles : sharedtransform/Quaternions to Rotation Angles  rotationOrder=ZYX  aMode=aMode
  Selector : Selector  InputPortWidth=3  IndexOptions=Index vector (dialog)  Indices=[3 2 1]  OutputSizes=1
  Selector1 : Selector  InputPortWidth=18  IndexOptions=Index vector (dialog)  Indices=[9]  OutputSizes=1
  Subsystem1 : Subsystem
  Subsystem2 : Subsystem
  Terminator{,1..4} (5 alike) : Terminator
  Transpose{,1..3} (4 alike) : Math  Operator=transpose
  Wrap To Zero1 : simulink/Discontinuities/Wrap To Zero  Threshold=1500
  timestamp : Outport
  Bus Element Out : Outport  Port=2  PortName=State  Element=position_inertial
  Bus Element Out1 : Outport  Port=2  PortName=State  Element=velocity_inertial
  Bus Element Out2 : Outport  Port=2  PortName=State  Element=course
  Bus Element Out3 : Outport  Port=2  PortName=State  Element=gndSpeed
  Bus Element Out4 : Outport  Port=2  PortName=State  Element=velocity_body
  Bus Element Out5 : Outport  Port=2  PortName=State  Element=euler
  Bus Element Out6 : Outport  Port=2  PortName=State  Element=ypr
  Bus Element Out7 : Outport  Port=2  PortName=State  Element=quat
  Bus Element Out8 : Outport  Port=2  PortName=State  Element=pqr
  Bus Element Out9 : Outport  Port=2  PortName=State  Element=airspeed
  VTOL_Switch : Outport  Port=3
  wires:
  [arm] -> Subsystem1/1(Trigger)
  Bus Selector1/4 -> Mux1/1  "<vx>"
  Transpose2/1 -> Matrix Multiply/1
  PX4 uORB Read3/1 -> Terminator/1
  Bus Selector2/2 -> timestamp/1  "<timestamp>"
  PX4 uORB Read3/2 -> Bus Selector3/1
  Bus Selector/1 -> Data Type Conversion6/1  "<q>"
  PX4 uORB Read1/1 -> Terminator1/1
  Bus Selector1/5 -> Mux1/2  "<vy>"
  Mux1/1 -> Data Type Conversion4/1  "x"
  Bus Selector1/6 -> Mux1/3  "<vz>"
  Mux/1 -> Data Type Conversion5/1
  Bus Selector1/1 -> Mux/1  "<x>"
  Transpose1/1 -> Coordinate Transformation Conversion/1
  PX4 uORB Read/1 -> Terminator2/1
  Data Type Conversion2/1 -> Transpose3/1
  MATLAB Function/1(y) -> Transpose1/1, Bus Element Out7/1, Quaternions to Rotation Angles/1, Transpose/1
  Bus Selector3/1 -> Data Type Conversion10/1  "<true_airspeed_m_s>"
  Quaternions to Rotation Angles/1 -> Subsystem1/2(Varying YPR Measurement)
  Data Type Conversion5/1 -> Subsystem2/2(Varying XYZ Measurement)
  PX4 uORB Read2/1 -> Terminator3/1
  Transpose3/1 -> Data Type Conversion1/1
  Subsystem1/1(Adjusted YPR Measurement) -> Data Type Conversion9/1
  Bus Selector1/3 -> Mux/3  "<z>"
  Transpose/1 -> Coordinate Transformation Conversion1/1
  PX4 uORB Read2/2 -> Bus Selector2/1
  [arm] -> Subsystem2/1(Trigger)
  Coordinate Transformation Conversion/1 -> Selector/1
  Bus Selector1/2 -> Mux/2  "<y>"
  Coordinate Transformation Conversion1/1 -> Matrix Multiply/2
  [velocity_inertial] -> Transpose2/1
  Selector/1 -> Data Type Conversion7/1
  Bus Selector2/1 -> Data Type Conversion2/1  "<xyz>"
  Matrix Multiply/1 -> Data Type Conversion3/1
  Subsystem2/1(Adjusted XYZ Measurement) -> Bus Element Out/1
  Input/1 -> [arm]
  PX4 uORB Read1/2 -> Bus Selector1/1
  PX4 uORB Read/2 -> Bus Selector/1
  Data Type Conversion4/1 -> [velocity_inertial], Bus Element Out1/1, MATLAB Function1/1(vxyz)
  Data Type Conversion6/1 -> MATLAB Function/1(u)
  MATLAB Function1/1(course) -> Bus Element Out2/1
  MATLAB Function1/2(gndSpeed) -> Bus Element Out3/1
  Data Type Conversion3/1 -> Bus Element Out4/1
  Data Type Conversion7/1 -> Bus Element Out5/1
  Data Type Conversion9/1 -> Bus Element Out6/1
  Data Type Conversion1/1 -> Bus Element Out8/1
  Data Type Conversion10/1 -> Bus Element Out9/1
  Selector1/1 -> Wrap To Zero1/1
  PX4 uORB Read4/2 -> Bus Selector4/1
  Bus Selector4/1 -> Selector1/1  "<values>"
  PX4 uORB Read4/1 -> Terminator4/1
  NOT1/1 -> VTOL_Switch/1
  Wrap To Zero1/1 -> NOT1/1

== system buildover_fullstatemachine/Subsystem3/Subsystem1 ==
  Trigger : Inport
  Varying YPR Measurement : Inport  Port=2
  Custom Single Sampler : Subsystem
  Demux : Demux  Outputs=3
  Mux3 : Mux  Inputs=3
  Sum : Sum  Inputs=|-+
  Adjusted YPR Measurement : Outport
  wires:
  Trigger/1 -> Custom Single Sampler/1(Trigger)
  Varying YPR Measurement/1 -> Demux/1, Custom Single Sampler/2(Varying Measurement)
  Custom Single Sampler/1("Initial Measurement ") -> Sum/1
  Demux/3 -> Mux3/3
  Sum/1 -> Mux3/1
  Demux/1 -> Sum/2
  Demux/2 -> Mux3/2
  Mux3/1 -> Adjusted YPR Measurement/1

== system buildover_fullstatemachine/Subsystem3/Subsystem2 ==
  Trigger : Inport
  Varying XYZ Measurement : Inport  Port=2
  Custom Single Sampler2 : Subsystem
  Demux : Demux  Outputs=3
  Mux3 : Mux  Inputs=3
  Adjusted XYZ Measurement : Outport
  wires:
  Trigger/1 -> Custom Single Sampler2/1(Trigger)
  Varying XYZ Measurement/1 -> Demux/1
  Mux3/1 -> Adjusted XYZ Measurement/1
  Demux/3 -> Custom Single Sampler2/2(Varying Measurement)
  Custom Single Sampler2/1("Adjusted Measurement ") -> Mux3/3
  Demux/1 -> Mux3/1
  Demux/2 -> Mux3/2

== system buildover_fullstatemachine/Subsystem3/Subsystem1/Custom Single Sampler ==
  Trigger : Inport
  Varying Measurement : Inport  Port=2
  Memory : Memory
  Sample and Hold : dspsigops/Sample and Hold  trig=Rising edge  initCond=0  latchinput=off
  Selector : Selector  InputPortWidth=3  IndexOptions=Index vector (dialog)  Indices=[1]  OutputSizes=1
  "Initial Measurement " : Outport
  wires:
  Sample and Hold/1 -> "Initial Measurement "/1
  Trigger/1 -> Memory/1
  Varying Measurement/1 -> Selector/1
  Selector/1 -> Sample and Hold/1
  Memory/1 -> Sample and Hold/Trigger

== system buildover_fullstatemachine/Subsystem3/Subsystem2/Custom Single Sampler2 ==
  Trigger : Inport
  Varying Measurement : Inport  Port=2
  Memory : Memory
  Sample and Hold : dspsigops/Sample and Hold  trig=Rising edge  initCond=0  latchinput=off
  Sum : Sum  Inputs=|-+
  "Adjusted Measurement " : Outport
  wires:
  Trigger/1 -> Memory/1
  Varying Measurement/1 -> Sum/2, Sample and Hold/1
  Memory/1 -> Sample and Hold/Trigger
  Sample and Hold/1 -> Sum/1
  Sum/1 -> "Adjusted Measurement "/1

== matlab function buildover_fullstatemachine/Subsystem3/MATLAB Function1 ==
  data: vxyz input; course output; gndSpeed output
function [course, gndSpeed] = fcn(vxyz)
    vx = vxyz(1);
    vy = vxyz(2);

    course = atan2(vy, vx);
    gndSpeed = norm([vx, vy]);
end

== matlab function buildover_fullstatemachine/Subsystem3/MATLAB Function ==
  data: u input; y output
function y = fcn(u)
    if any(isnan(u))
        y = [1 0 0 0];
    elseif norm(u) < 0.1
        y = [1 0 0 0];
    else
        y = u/norm(u);
    end
end

== stateflow chart buildover_fullstatemachine/Chart ==
  state off_disarmed
  state Rotor_Spin_Up
  state off_armed
  state VTOL
  state Rotor_ACCEL
  state Kill
  state Quad_Hover
  state Rotor_DEACCEL_prep
  state Rotor_DEACCEL
  state FF_Preparation
  state Forward_Flight
  Rotor_ACCEL -> Rotor_DEACCEL_prep [order 2] : [btn_state == 2 | btn_state  == 6]
  Rotor_ACCEL -> VTOL [order 1] : [a_rotor == 0]
  (default) -> off_disarmed
  Rotor_DEACCEL -> off_disarmed [order 2] : [btn_state == 7 & a_rotor == 0]
  Quad_Hover -> off_disarmed [order 2] : [btn_state == 7]
  off_disarmed -> Kill [order 2] : [kill_state == 1]
  Kill -> off_disarmed : [kill_state == 0 & arm_state == 0]
  off_armed -> off_disarmed [order 3] : [arm_state == 0]
  off_disarmed -> off_armed [order 1] : [arm_state == 1 & btn_state == 1]
  off_armed -> Rotor_Spin_Up [order 2] : [btn_state == 4]
  Rotor_Spin_Up -> VTOL [order 2] : [a_rotor == 0]
  Rotor_Spin_Up -> Kill [order 1] : [kill_state == 1]
  off_armed -> Quad_Hover [order 1] : [btn_state == 2]
  off_armed -> Kill [order 4] : [kill_state == 1]
  VTOL -> Rotor_DEACCEL_prep [order 2] : [btn_state == 2 | btn_state == 6 | btn_state == 7]
  VTOL -> Kill [order 1] : [kill_state == 1]
  Rotor_ACCEL -> Kill [order 3] : [kill_state == 1]
  Quad_Hover -> Rotor_ACCEL [order 1] : [btn_state == 4]
  Rotor_DEACCEL_prep -> Kill [order 1] : [kill_state == 1]
  Quad_Hover -> Kill [order 3] : [kill_state == 1]
  Rotor_DEACCEL -> Quad_Hover [order 3] : [btn_state == 2 & a_rotor == 0]
  Rotor_DEACCEL -> Kill [order 1] : [kill_state == 1]
  Forward_Flight -> Kill [order 1] : [kill_state == 1]
  FF_Preparation -> Kill [order 1] : [kill_state == 1]
  FF_Preparation -> Quad_Hover [order 2] : [btn_state == 2]
  Quad_Hover -> FF_Preparation [order 4] : [btn_state == 6]
  Rotor_DEACCEL_prep -> Rotor_DEACCEL [order 2] : [abs(rcbangle_speed) < 100 & abs(lcbangle_speed) < 100]
  FF_Preparation -> Forward_Flight [order 3] : [px4_vtolswitch == 1 & abs(rcbangle_speed) < 100 & abs(lcbangle_speed) < 100]
  Forward_Flight -> FF_Preparation [order 2] : [px4_vtolswitch == 0]
  Rotor_DEACCEL -> FF_Preparation [order 4] : [btn_state == 6 & a_rotor == 0]
  data: sf_internal_action_state_placeholder_data local double size=1 =0; sf_internal_action_state_placeholder_data local double size=1 =0; sf_internal_action_state_placeholder_data local double size=1 =0; sf_internal_action_state_placeholder_data local double size=1 =0; sf_internal_action_state_placeholder_data local double size=1 =0; sf_internal_action_state_placeholder_data local double size=1 =0; sf_internal_action_state_placeholder_data local double size=1 =0; sf_internal_action_state_placeholder_data local double size=1 =0; sf_internal_action_state_placeholder_data local double size=1 =0; sf_internal_action_state_placeholder_data local double size=1 =0; sf_internal_action_state_placeholder_data local double size=1 =0; arm_state input; lcb_speed output; leftcb_angle output; mainrotor_control output; rcb_speed output; rightcb_angle output; slider_position output; kill_state input; btn_state input; a_rotor input; w_ff_gain output; tau_ff_gain output; Tune_ID output; lcbangle_speed input; rcbangle_speed input; arm_output output; px4_vtolswitch input; des_vx input
